simulink model "Closed_Loop_Q12"  (R2016b)
settings: Solver=VariableStepAuto  StartTime=0.0  StopTime=40  RelTol=1e-3
settings Model: Creator=Yazdanpanah  LastModifiedBy=fatae
settings DataIOCC: ReturnWorkspaceOutputs=on
settings SFSimCC: SimUseLocalCustomCode=on
settings RTWCC: RTWUseLocalCustomCode=on

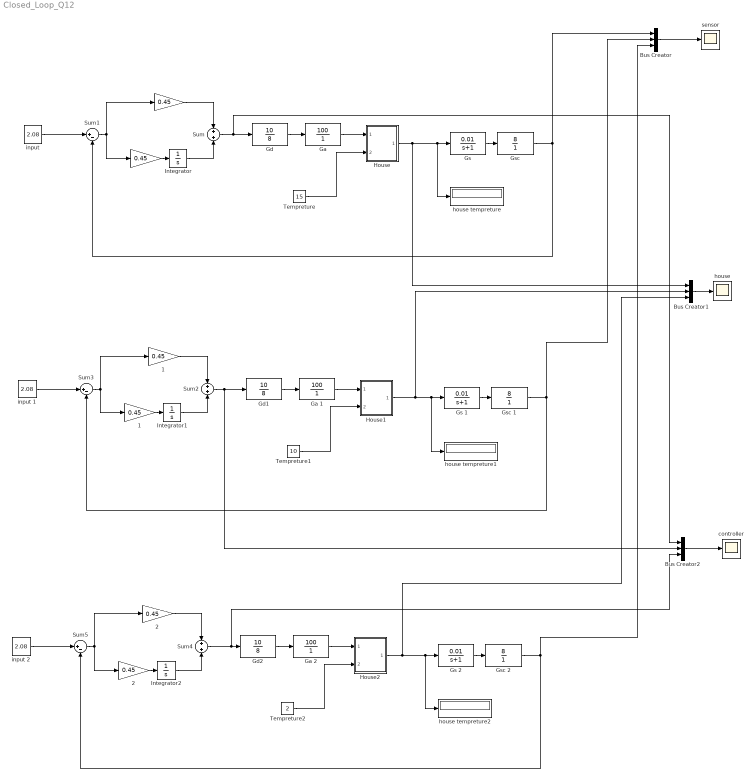
== system Closed_Loop_Q12 ==
   {,,1,1..2,2} (6 alike) : Gain  Gain=0.45
  Bus Creator : BusCreator  Inputs=3
  Bus Creator1 : BusCreator  Inputs=3
  Bus Creator2 : BusCreator  Inputs=3
  "Ga " : TransferFcn  Numerator=[100]  Denominator=[0 1]
  Ga 1 : TransferFcn  Numerator=[100]  Denominator=[0 1]
  Ga 2 : TransferFcn  Numerator=[100]  Denominator=[0 1]
  Gd : TransferFcn  Numerator=[10]  Denominator=[0 8]
  Gd1 : TransferFcn  Numerator=[10]  Denominator=[0 8]
  Gd2 : TransferFcn  Numerator=[10]  Denominator=[0 8]
  "Gs " : TransferFcn  Numerator=[0.01]  Denominator=[1 1]
  Gs 1 : TransferFcn  Numerator=[0.01]  Denominator=[1 1]
  Gs 2 : TransferFcn  Numerator=[0.01]  Denominator=[1 1]
  "Gsc " : TransferFcn  Numerator=[8]  Denominator=[0 1]
  Gsc 1 : TransferFcn  Numerator=[8]  Denominator=[0 1]
  Gsc 2 : TransferFcn  Numerator=[8]  Denominator=[0 1]
  House : Subsystem
      mask Display: image(fullfile(matlabroot,'toolbox','simulink','simdemos','simgeneral','images','HouseHeatHousePix.svg'))
  House1 : Subsystem
      mask Display: image(fullfile(matlabroot,'toolbox','simulink','simdemos','simgeneral','images','HouseHeatHousePix.svg'))
  House2 : Subsystem
      mask Display: image(fullfile(matlabroot,'toolbox','simulink','simdemos','simgeneral','images','HouseHeatHousePix.svg'))
  Integrator : Integrator
  Integrator1 : Integrator
  Integrator2 : Integrator
  Sum : Sum
  Sum1 : Sum  Inputs=|+-
  Sum2 : Sum
  Sum3 : Sum  Inputs=|+-
  Sum4 : Sum
  Sum5 : Sum  Inputs=|+-
  Tempreture : Constant  Value=15
  Tempreture1 : Constant  Value=10
  Tempreture2 : Constant  Value=2
  controller : Scope
  house : Scope
  house tempreture : Display
  house tempreture1 : Display
  house tempreture2 : Display
  "input " : Constant  Value=2.08
  input 1 : Constant  Value=2.08
  input 2 : Constant  Value=2.08
  sensor : Scope
  wires:
  Sum/1 -> Bus Creator2/1, Gd/1
  "Gsc "/1 -> Bus Creator/1, Sum1/2
  Bus Creator/1 -> sensor/1
  Sum1/1 -> " "/1, " "/1
  Integrator/1 -> Sum/2
  " "/1 -> Integrator/1
  House/1(Room Temp Troom) -> Bus Creator1/1, "Gs "/1, house tempreture/1
  Gd/1 -> "Ga "/1
  "Gs "/1 -> "Gsc "/1
  Tempreture/1 -> House/2(Outdoor Temp Tout)
  "input "/1 -> Sum1/1
  "Ga "/1 -> House/1(Heater QDot In)
  " "/1 -> Sum/1
  Sum2/1 -> Bus Creator2/2, Gd1/1
  Bus Creator1/1 -> house/1
  Sum3/1 -> " 1"/1, " 1"/1
  Integrator1/1 -> Sum2/2
  " 1"/1 -> Integrator1/1
  House1/1(Room Temp Troom) -> Bus Creator1/2, Gs 1/1, house tempreture1/1
  Gd1/1 -> Ga 1/1
  Gs 1/1 -> Gsc 1/1
  Tempreture1/1 -> House1/2(Outdoor Temp Tout)
  input 1/1 -> Sum3/1
  Ga 1/1 -> House1/1(Heater QDot In)
  " 1"/1 -> Sum2/1
  Sum4/1 -> Bus Creator2/3, Gd2/1
  Gsc 2/1 -> Bus Creator/3, Sum5/2
  Bus Creator2/1 -> controller/1
  Sum5/1 -> " 2"/1, " 2"/1
  Integrator2/1 -> Sum4/2
  " 2"/1 -> Integrator2/1
  House2/1(Room Temp Troom) -> Bus Creator1/3, Gs 2/1, house tempreture2/1
  Gd2/1 -> Ga 2/1
  Gs 2/1 -> Gsc 2/1
  Tempreture2/1 -> House2/2(Outdoor Temp Tout)
  input 2/1 -> Sum5/1
  Ga 2/1 -> House2/1(Heater QDot In)
  " 2"/1 -> Sum4/1
  Gsc 1/1 -> Bus Creator/2, Sum3/2

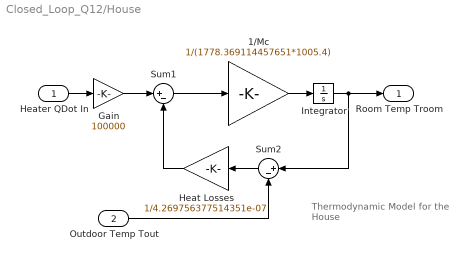
== system Closed_Loop_Q12/House ==
  note: Thermodynamic Model
      | for the House
  Heater QDot In : Inport
  Outdoor Temp Tout : Inport  Port=2
  1/Mc : Gain  Gain=1/(1778.369114457651*1005.4)  SaturateOnIntegerOverflow=on  OutDataTypeStr=Inherit: Same as input  ParamDataTypeStr=Inherit: Same as input
  Gain : Gain  Gain=100000
  Heat Losses : Gain  Gain=1/4.269756377514351e-07  SaturateOnIntegerOverflow=on  OutDataTypeStr=Inherit: Same as input  ParamDataTypeStr=Inherit: Same as input
  Integrator : Integrator  InitialCondition=20
  Sum1 : Sum  Inputs=|+-  SaturateOnIntegerOverflow=on  InputSameDT=on  OutDataTypeStr=Inherit: Same as first input
  Sum2 : Sum  Inputs=|+-  SaturateOnIntegerOverflow=on  InputSameDT=on  OutDataTypeStr=Inherit: Same as first input
  Room Temp Troom : Outport  InitialOutput=0
  wires:
  Outdoor Temp Tout/1 -> Sum2/2
  Heater QDot In/1 -> Gain/1
  Sum1/1 -> 1/Mc/1
  Sum2/1 -> Heat Losses/1
  Heat Losses/1 -> Sum1/2
  1/Mc/1 -> Integrator/1
  Integrator/1 -> Sum2/1, Room Temp Troom/1
  Gain/1 -> Sum1/1

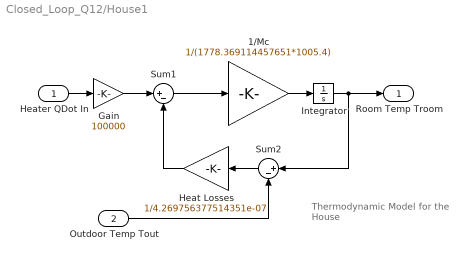
== system Closed_Loop_Q12/House1 ==
  note: Thermodynamic Model
      | for the House
  Heater QDot In : Inport
  Outdoor Temp Tout : Inport  Port=2
  1/Mc : Gain  Gain=1/(1778.369114457651*1005.4)  SaturateOnIntegerOverflow=on  OutDataTypeStr=Inherit: Same as input  ParamDataTypeStr=Inherit: Same as input
  Gain : Gain  Gain=100000
  Heat Losses : Gain  Gain=1/4.269756377514351e-07  SaturateOnIntegerOverflow=on  OutDataTypeStr=Inherit: Same as input  ParamDataTypeStr=Inherit: Same as input
  Integrator : Integrator  InitialCondition=20
  Sum1 : Sum  Inputs=|+-  SaturateOnIntegerOverflow=on  InputSameDT=on  OutDataTypeStr=Inherit: Same as first input
  Sum2 : Sum  Inputs=|+-  SaturateOnIntegerOverflow=on  InputSameDT=on  OutDataTypeStr=Inherit: Same as first input
  Room Temp Troom : Outport  InitialOutput=0
  wires:
  Outdoor Temp Tout/1 -> Sum2/2
  Heater QDot In/1 -> Gain/1
  Sum1/1 -> 1/Mc/1
  Sum2/1 -> Heat Losses/1
  Heat Losses/1 -> Sum1/2
  1/Mc/1 -> Integrator/1
  Integrator/1 -> Sum2/1, Room Temp Troom/1
  Gain/1 -> Sum1/1

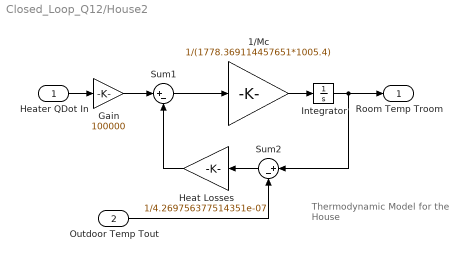
== system Closed_Loop_Q12/House2 ==
  note: Thermodynamic Model
      | for the House
  Heater QDot In : Inport
  Outdoor Temp Tout : Inport  Port=2
  1/Mc : Gain  Gain=1/(1778.369114457651*1005.4)  SaturateOnIntegerOverflow=on  OutDataTypeStr=Inherit: Same as input  ParamDataTypeStr=Inherit: Same as input
  Gain : Gain  Gain=100000
  Heat Losses : Gain  Gain=1/4.269756377514351e-07  SaturateOnIntegerOverflow=on  OutDataTypeStr=Inherit: Same as input  ParamDataTypeStr=Inherit: Same as input
  Integrator : Integrator  InitialCondition=20
  Sum1 : Sum  Inputs=|+-  SaturateOnIntegerOverflow=on  InputSameDT=on  OutDataTypeStr=Inherit: Same as first input
  Sum2 : Sum  Inputs=|+-  SaturateOnIntegerOverflow=on  InputSameDT=on  OutDataTypeStr=Inherit: Same as first input
  Room Temp Troom : Outport  InitialOutput=0
  wires:
  Outdoor Temp Tout/1 -> Sum2/2
  Heater QDot In/1 -> Gain/1
  Sum1/1 -> 1/Mc/1
  Sum2/1 -> Heat Losses/1
  Heat Losses/1 -> Sum1/2
  1/Mc/1 -> Integrator/1
  Integrator/1 -> Sum2/1, Room Temp Troom/1
  Gain/1 -> Sum1/1
